simulink model "dont_enter_at_initialization"  (Simulink 6.6)
settings: Solver=FixedStepDiscrete  StartTime=0.0  StopTime=10.0  FixedStep=1  RelTol=1e-3
settings Model: Creator=vBuskirk  LastModifiedBy=vBuskirk

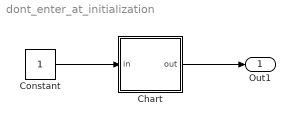
== system dont_enter_at_initialization ==
  Chart : Stateflow chart
  Constant : Constant
  Out1 : Outport
  wires:
  Constant/1 -> Chart/1(in)
  Chart/1(out) -> Out1/1

== stateflow chart Chart ==
  state s1
  state s2
  s1 -> s2 : / out = in;
  (default) -> s1
  data: in input inherited; out output double
